simulink model "sys_2"  (R2017a)
settings: Solver=FixedStepAuto  StartTime=0.0  StopTime=40  FixedStep=0.005  RelTol=1e-3
values from neighbouring files (symbols this model uses):
  B = [b -b;-b b]    [OBS_CONT.m]    (also in OBS_CONT_MORE_STIFF.m)
  D = zeros(1,1)    [OBS_CONT.m]
  F = [0 1 0 0;-k/j2 -b/j2 k/j2 b/j2;0 0 0 01;k/j1 b/j1 -k/j1 -b/j1]    [OBS_CONT.m]
  G = [0;0;0;1/j1]    [OBS_CONT.m]
  H = [1 0 0 0]    [OBS_CONT.m]
  Kc = [-0.26139 0.041515 0.65538 1.1604]    [OBS_CONT.m]    (also in OBS_CONT_MORE_STIFF.m = place(F,G,p_cont))
  Ke = [22.0004 242.0531 1512.84032 5485.9822]'    [OBS_CONT.m]    (also in OBS_CONT_MORE_STIFF.m = Ke')
undefined symbols (not defined in the file or in its folder): A, A_c, B_c, C, C_c, V, V_c
settings Model: Creator=ASUS  LastModifiedBy=ASUS

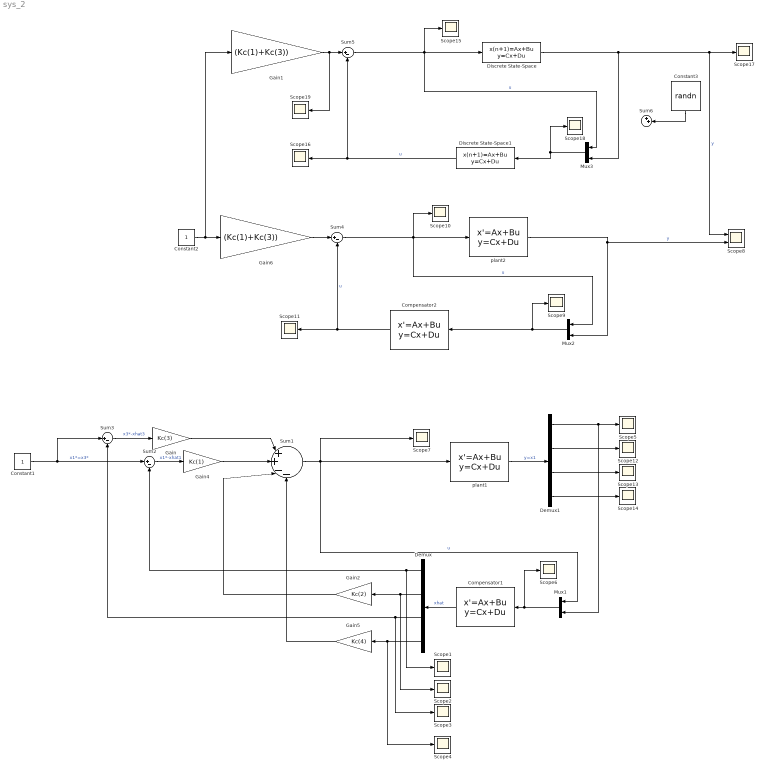
== system sys_2 ==
  Compensator1 : StateSpace  A=F-Ke*H  B=[G Ke]  C=[1 0 0 0;0 1 0 0;0 0 1 0;0 0 0 1]  D=[0 0;0 0;0 0;0 0]  X0=0
  Compensator2 : StateSpace  A=F-Ke*H  B=[G Ke]  C=Kc  D=[D D]  X0=0
  Constant1 : Constant
  Constant2 : Constant
  Constant3 : Constant  Value=randn
  Demux : Demux
  Demux1 : Demux
  Discrete State-Space : DiscreteStateSpace  A=A  B=B  C=C  D=V  SampleTime=0.01
  Discrete State-Space1 : DiscreteStateSpace  A=A_c  B=B_c  C=C_c  D=V_c  SampleTime=0.01
  Gain : Gain  Gain=Kc(3)
  Gain1 : Gain  Gain=(Kc(1)+Kc(3))
  Gain2 : Gain  Gain=Kc(2)
  Gain4 : Gain  Gain=Kc(1)
  Gain5 : Gain  Gain=Kc(4)
  Gain6 : Gain  Gain=(Kc(1)+Kc(3))
  Mux1 : Mux  Inputs=2
  Mux2 : Mux  Inputs=2
  Mux3 : Mux  Inputs=2
  Scope{1..7,9..19} (18 alike) : Scope
  Scope8 : Scope  NumInputPorts=2
  Sum1 : Sum  Inputs=|++--
  Sum{2..5} (4 alike) : Sum  Inputs=|+-
  Sum6 : Sum  Inputs=|++
  plant1 : StateSpace  A=F  B=G  C=[1 0 0 0;0 1 0 0;0 0 1 0;0 0 0 1]  D=[0;0;0;0]  X0=0
  plant2 : StateSpace  A=F  B=G  C=H  D=D  X0=0
  wires:
  Mux1/1 -> Scope6/1, Compensator1/1
  Sum1/1 -> Scope7/1, Mux1/1, plant1/1  "u"
  Compensator1/1 -> Demux/1  "xhat"
  Demux/1 -> Scope1/1, Sum2/2
  Gain2/1 -> Sum1/3
  Demux/3 -> Scope3/1, Sum3/2
  Demux/2 -> Scope2/1, Gain2/1
  Gain4/1 -> Sum1/2
  Sum2/1 -> Gain4/1  "x1*-xhat1"
  Constant1/1 -> Sum3/1, Sum2/1  "x1*=x3*"
  Sum3/1 -> Gain/1  "x3*-xhat3"
  Demux/4 -> Scope4/1, Gain5/1
  Gain/1 -> Sum1/1
  Constant2/1 -> Gain1/1, Gain6/1
  Sum4/1 -> Scope10/1, Mux2/1, plant2/1  "u"
  plant2/1 -> Mux2/2, Scope8/2  "y"
  Mux2/1 -> Scope9/1, Compensator2/1
  Compensator2/1 -> Sum4/2, Scope11/1  "u"
  Gain6/1 -> Sum4/1
  Gain5/1 -> Sum1/4
  plant1/1 -> Demux1/1  "y=x1"
  Demux1/1 -> Scope5/1, Mux1/2
  Demux1/3 -> Scope13/1
  Demux1/4 -> Scope14/1
  Demux1/2 -> Scope12/1
  Gain1/1 -> Scope19/1, Sum5/1
  Discrete State-Space1/1 -> Sum5/2, Scope16/1  "u"
  Sum5/1 -> Mux3/1, Discrete State-Space/1, Scope15/1  "u"
  Mux3/1 -> Discrete State-Space1/1, Scope18/1
  Discrete State-Space/1 -> Scope8/1, Scope17/1, Mux3/2  "y"
  Constant3/1 -> Sum6/2
